simulink model "fil_videosharp_sim"  (R2018b)
settings: Solver=FixedStepDiscrete  StartTime=0.0  StopTime=inf  RelTol=1e-3
InitFcn:
  | filter = fi(fspecial('unsharp'),1,16,12);
  | 
  | % video size excluding the blanking periods
  | fileName = get_param('fil_videosharp_sim/From Multimedia File',  'inputFilename');
  | x=mmfileinfo(fileName);
  | v = x.Video ;
  | H = v.Height;
  | W = v.Width;
  | %H = 176;
  | %W = 240;
  | activeVideoSize = [H W];
  | 
  | % horizontal and vertical blanking
  | hBlanking = 0;
  | vBlanking = 0;
undefined symbols (not defined in the file): gcbh, gray, none, NumBits1, NumBits2, Rec, SDTV, Slope1, Slope2, videoinput
libraries: simulink x19, visionconversions x3, dspsigattribs x3, visiongeotforms x3, dspbuff3 x3, hdlsllib x3, visionsinks x1, dspvision x1, imaqlib x1, simulink_need_slupdate x1, fillib x1
(part 3 of 3)

== system fil_videosharp_sim/Streaming 2-D FIR Filter/Line Memory/Line Memory Controller/Write Col Counter ==
  enable : Inport
  reload : Inport  Port=2
  DataTypeConversion : DataTypeConversion  OutDataTypeStr=fixdt(SIGN==1,((WLTYPE==1) * ( ceil(log2(MAX_VAL-MIN_VAL+1)) + double(SIGN==1) ) ) + ((WLTYPE~=1)* WL ),0)
  Unit Delay : UnitDelay  InitialCondition=INIT_VAL  SampleTime=-1
  eML Counter : MATLAB Function  TreatAsAtomicUnit=on
  count : Outport
  wires:
  DataTypeConversion/1 -> Unit Delay/1
  eML Counter/1(nextCount) -> DataTypeConversion/1
  Unit Delay/1 -> eML Counter/1(currentCount), count/1
  reload/1 -> eML Counter/3(reload)
  enable/1 -> eML Counter/2(enb)

== system fil_videosharp_sim/Streaming 2-D FIR Filter/Line Memory/Line Memory Controller/Write Line Counter ==
  enable : Inport
  reload : Inport  Port=2
  DataTypeConversion : DataTypeConversion  OutDataTypeStr=fixdt(SIGN==1,((WLTYPE==1) * ( ceil(log2(MAX_VAL-MIN_VAL+1)) + double(SIGN==1) ) ) + ((WLTYPE~=1)* WL ),0)
  Unit Delay : UnitDelay  InitialCondition=INIT_VAL  SampleTime=-1
  eML Counter : MATLAB Function  TreatAsAtomicUnit=on
  count : Outport
  wires:
  enable/1 -> eML Counter/2(enb)
  reload/1 -> eML Counter/3(reload)
  Unit Delay/1 -> eML Counter/1(currentCount), count/1
  eML Counter/1(nextCount) -> DataTypeConversion/1
  DataTypeConversion/1 -> Unit Delay/1

== system fil_videosharp_sim/Streaming 2-D FIR Filter/Line Memory/Line Memory Controller/zzzz1 ==

== system fil_videosharp_sim/Streaming 2-D FIR Filter/Line Memory/Line Memory Controller/zzzz3 ==

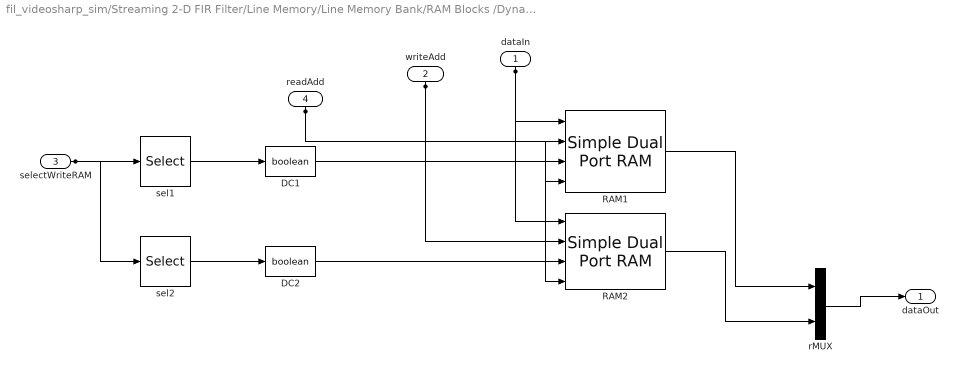
== system fil_videosharp_sim/Streaming 2-D FIR Filter/Line Memory/Line Memory Bank/RAM Blocks /Dynamic RAM Blocks ==
  dataIn : Inport
  writeAdd : Inport  Port=2
  selectWriteRAM : Inport  Port=3
  readAdd : Inport  Port=4
  DC1 : DataTypeConversion  OutDataTypeStr=boolean
  DC2 : DataTypeConversion  OutDataTypeStr=boolean
  RAM1 : hdlsllib/HDL RAMs/Simple Dual Port RAM  ram_size=WL
      settings: SourceProductName=HDL Coder  SourceProductBaseCode=HD
  RAM2 : hdlsllib/HDL RAMs/Simple Dual Port RAM  ram_size=WL
      settings: SourceProductName=HDL Coder  SourceProductBaseCode=HD
  rMUX : Mux  Inputs=2
  sel1 : Selector  InputPortWidth=2  IndexOptions=Index vector (dialog)  Indices=[1]  OutputSizes=1
  sel2 : Selector  InputPortWidth=2  IndexOptions=Index vector (dialog)  Indices=[2]  OutputSizes=1
  dataOut : Outport
  wires:
  selectWriteRAM/1 -> sel1/1, sel2/1
  sel1/1 -> DC1/1
  DC1/1 -> RAM1/3
  dataIn/1 -> RAM1/1, RAM2/1
  writeAdd/1 -> RAM1/2, RAM2/2
  readAdd/1 -> RAM1/4, RAM2/4
  RAM1/1 -> rMUX/1
  sel2/1 -> DC2/1
  DC2/1 -> RAM2/3
  RAM2/1 -> rMUX/2
  rMUX/1 -> dataOut/1

== system fil_videosharp_sim/Streaming 2-D FIR Filter/Line Memory/Line Memory Controller/Adjust Sync Signals/Detect Frame End ==
  lineEnd : Inport
  frameHeight : Inport  Port=2
  rowIndex : Inport  Port=3
  AND1 : Logic  IconShape=distinctive  AllPortsSameDT=off  OutDataTypeStr=boolean
  Add : Sum
  Constant2 : Constant  OutDataTypeStr=Inherit: Inherit via back propagation
  Relational Operator : RelationalOperator  Operator===  OutDataTypeStr=boolean  RndMeth=Nearest
  valid : Outport
  wires:
  Constant2/1 -> Add/1
  Add/1 -> Relational Operator/2
  Relational Operator/1 -> AND1/2
  lineEnd/1 -> AND1/1
  rowIndex/1 -> Add/2
  frameHeight/1 -> Relational Operator/1
  AND1/1 -> valid/1

== system fil_videosharp_sim/Streaming 2-D FIR Filter/Line Memory/Line Memory Controller/Adjust Sync Signals/Detect Frame Start ==
  lineStart : Inport
  rowIndex : Inport  Port=2
  AND1 : Logic  IconShape=distinctive  AllPortsSameDT=off  OutDataTypeStr=boolean
  Compare To Constant1 : simulink/Logic and Bit Operations/Compare To Constant  relop===  const=0  OutDataTypeStr=boolean  ZeroCross=off
  alignedFrameStart : Outport
  wires:
  AND1/1 -> alignedFrameStart/1
  rowIndex/1 -> Compare To Constant1/1
  lineStart/1 -> AND1/1
  Compare To Constant1/1 -> AND1/2

== system fil_videosharp_sim/Streaming 2-D FIR Filter/Line Memory/Line Memory Controller/Adjust Sync Signals/Detect Line End ==
  dataValidOut : Inport
  frameWidth : Inport  Port=2
  colIndex : Inport  Port=3
  AND1 : Logic  IconShape=distinctive  AllPortsSameDT=off  OutDataTypeStr=boolean
  Add : Sum
  Constant2 : Constant  OutDataTypeStr=Inherit: Inherit via back propagation
  Relational Operator : RelationalOperator  Operator===  OutDataTypeStr=boolean  RndMeth=Nearest
  lineEnd : Outport
  wires:
  AND1/1 -> lineEnd/1
  frameWidth/1 -> Relational Operator/1
  colIndex/1 -> Add/2
  dataValidOut/1 -> AND1/1
  Relational Operator/1 -> AND1/2
  Add/1 -> Relational Operator/2
  Constant2/1 -> Add/1

== system fil_videosharp_sim/Streaming 2-D FIR Filter/Line Memory/Line Memory Controller/Adjust Sync Signals/Detect Line Start ==
  dataValidOut : Inport
  colIndex : Inport  Port=2
  AND1 : Logic  AllPortsSameDT=off  OutDataTypeStr=boolean
  Compare To Constant1 : simulink/Logic and Bit Operations/Compare To Constant  relop===  const=0  OutDataTypeStr=boolean  ZeroCross=off
  alignedLineStart : Outport
  wires:
  Compare To Constant1/1 -> AND1/2
  dataValidOut/1 -> AND1/1
  colIndex/1 -> Compare To Constant1/1
  AND1/1 -> alignedLineStart/1

== system fil_videosharp_sim/Streaming 2-D FIR Filter/Line Memory/Line Memory Controller/Adjust Sync Signals/SyncMux ==
  activePixel : Inport
  lineStart : Inport  Port=2
  lineEnd : Inport  Port=3
  FrameStart : Inport  Port=4
  FrameEnd : Inport  Port=5
  Mux : Mux  Inputs=5
  syncOut : Outport
  wires:
  Mux/1 -> syncOut/1
  FrameEnd/1 -> Mux/5
  FrameStart/1 -> Mux/4
  lineEnd/1 -> Mux/3
  lineStart/1 -> Mux/2
  activePixel/1 -> Mux/1

== system fil_videosharp_sim/Streaming 2-D FIR Filter/Line Memory/Line Memory Controller/Read Control/Hold Valid Counter ==
  enable : Inport
  reload : Inport  Port=2
  DataTypeConversion : DataTypeConversion  OutDataTypeStr=fixdt(SIGN==1,((WLTYPE==1) * ( ceil(log2(MAX_VAL-MIN_VAL+1)) + double(SIGN==1) ) ) + ((WLTYPE~=1)* WL ),0)
  Unit Delay : UnitDelay  InitialCondition=INIT_VAL  SampleTime=-1
  eML Counter : MATLAB Function  TreatAsAtomicUnit=on
  count : Outport
  wires:
  enable/1 -> eML Counter/2(enb)
  reload/1 -> eML Counter/3(reload)
  Unit Delay/1 -> eML Counter/1(currentCount), count/1
  eML Counter/1(nextCount) -> DataTypeConversion/1
  DataTypeConversion/1 -> Unit Delay/1

== system fil_videosharp_sim/Streaming 2-D FIR Filter/Line Memory/Line Memory Controller/Read Control/Pos Edge Detect ==
  x : Inport
  Logical Operator1 : Logic  AllPortsSameDT=off  OutDataTypeStr=boolean
  Logical Operator2 : Logic  Operator=NOT  AllPortsSameDT=off  OutDataTypeStr=boolean
  Unit Delay1 : UnitDelay  SampleTime=-1
  y : Outport
  wires:
  x/1 -> Logical Operator1/1, Unit Delay1/1
  Logical Operator1/1 -> y/1
  Logical Operator2/1 -> Logical Operator1/2
  Unit Delay1/1 -> Logical Operator2/1

== system fil_videosharp_sim/Streaming 2-D FIR Filter/Line Memory/Line Memory Controller/Read Control/Pos Edge Detect1 ==
  x : Inport
  Logical Operator1 : Logic  AllPortsSameDT=off  OutDataTypeStr=boolean
  Logical Operator2 : Logic  Operator=NOT  AllPortsSameDT=off  OutDataTypeStr=boolean
  Unit Delay1 : UnitDelay  SampleTime=-1
  y : Outport
  wires:
  x/1 -> Logical Operator1/1, Unit Delay1/1
  Logical Operator1/1 -> y/1
  Logical Operator2/1 -> Logical Operator1/2
  Unit Delay1/1 -> Logical Operator2/1

== system fil_videosharp_sim/Streaming 2-D FIR Filter/Line Memory/Line Memory Controller/Read Control/Repeat Counter ==
  enable : Inport
  reload : Inport  Port=2
  DataTypeConversion : DataTypeConversion  OutDataTypeStr=fixdt(SIGN==1,((WLTYPE==1) * ( ceil(log2(MAX_VAL-MIN_VAL+1)) + double(SIGN==1) ) ) + ((WLTYPE~=1)* WL ),0)
  Unit Delay : UnitDelay  InitialCondition=INIT_VAL  SampleTime=-1
  eML Counter : MATLAB Function  TreatAsAtomicUnit=on
  count : Outport
  wires:
  DataTypeConversion/1 -> Unit Delay/1
  eML Counter/1(nextCount) -> DataTypeConversion/1
  Unit Delay/1 -> eML Counter/1(currentCount), count/1
  reload/1 -> eML Counter/3(reload)
  enable/1 -> eML Counter/2(enb)

== system fil_videosharp_sim/Streaming 2-D FIR Filter/Line Memory/Line Memory Controller/Read Control/Time Distance ==
  repeat : Inport
  newLine : Inport  Port=2
  Time Distance : MATLAB Function  TreatAsAtomicUnit=on
  Unit Delay1 : UnitDelay  SampleTime=-1
  Unit Delay7 : UnitDelay  SampleTime=-1
  currentDistance : Outport
  lastDistance : Outport  Port=2
  wires:
  repeat/1 -> Time Distance/2(repeatPulse)
  Unit Delay1/1 -> Time Distance/4(fromLastDist), lastDistance/1
  Unit Delay7/1 -> Time Distance/3(fromDistCounter), currentDistance/1
  newLine/1 -> Time Distance/1(inputPulse)
  Time Distance/2(toLastDist) -> Unit Delay1/1  "current_dist"
  Time Distance/1(toDistCounter) -> Unit Delay7/1  "Last_dist"

== system fil_videosharp_sim/Streaming 2-D FIR Filter/Line Memory/Line Memory Controller/Read Control/zzzz1 ==

== system fil_videosharp_sim/Streaming 2-D FIR Filter/Line Memory/Line Memory Controller/Read Control/zzzz2 ==

== system fil_videosharp_sim/Streaming 2-D FIR Filter/Line Memory/Line Memory Controller/Read Control/zzzz3 ==

== system fil_videosharp_sim/Streaming 2-D FIR Filter/Line Memory/Line Memory Controller/Read Control/zzzz5 ==

== system fil_videosharp_sim/Streaming 2-D FIR Filter/Line Memory/Line Memory Controller/Read Line Count/Read Line Counter1 ==
  enable : Inport
  reload : Inport  Port=2
  loadVal : Inport  Port=3
  DataTypeConversion : DataTypeConversion  OutDataTypeStr=fixdt(SIGN==1,((WLTYPE==1) * ( ceil(log2(MAX_VAL-MIN_VAL+1)) + double(SIGN==1) ) ) + ((WLTYPE~=1)* WL ),0)
  Unit Delay : UnitDelay  InitialCondition=INIT_VAL  SampleTime=-1
  eML Counter : MATLAB Function  TreatAsAtomicUnit=on
  count : Outport
  wires:
  enable/1 -> eML Counter/2(enb)
  reload/1 -> eML Counter/3(reload)
  Unit Delay/1 -> eML Counter/1(currentCount), count/1
  eML Counter/1(nextCount) -> DataTypeConversion/1
  DataTypeConversion/1 -> Unit Delay/1
  loadVal/1 -> eML Counter/4(loadVal)

== matlab function fil_videosharp_sim/Frame to Stream/Produce Row-Major Organized Output (Dimensions will be flipped) ==
  data: u input; y output; isInputRowMajor parameter
function y = condTranspose(u, isInputRowMajor)
%#eml

if (isInputRowMajor)
    y = u;
else
    y = permute(u,[2,1]);
end

== matlab function fil_videosharp_sim/Streaming 2-D FIR Filter/Line Memory/Aligned Demux/Aligned Pulse ==
  settings: fimath=hdlfimath
  data: valid input; earlyPulse input; alignedPulse output
function alignedPulse = align(valid,earlyPulse)

persistent earlyPulse_reg;
if isempty(earlyPulse_reg)
    earlyPulse_reg = false;
end

alignedPulse= (earlyPulse_reg || earlyPulse) && valid;

if (earlyPulse && ~valid)
    earlyPulse_reg=true;
elseif (earlyPulse_reg || earlyPulse) && valid;
    earlyPulse_reg=false;
end

== matlab function fil_videosharp_sim/Stream to Frame/Generate Control Signals ==
  data: activePixel input; frameValid output; frameStart input; frameEnd input; enable output
function [frameValid, enable] = ctrlSigGen(activePixel, frameStart, ...
    frameEnd)
%#eml

persistent enableFlag; % turns on after vsync pulse was received

persistent frameEndWithDelay;

% initialize persistent vars
if isempty(enableFlag)
   enableFlag = false; 
end

if isempty(frameEndWithDelay)
   frameEndWithDelay = false; 
end

if frameStart ~= 0
    enableFlag = true;
end

enable = frameEndWithDelay || activePixel;

frameValid =  frameEndWithDelay;


% Delay line block used to accumulate full frame has an inherent
% latency of 1.  We accommodate it by using a delayed version of 
% frameEnd signal in computing the enableFlag
frameEndWithDelay = frameEnd;

== matlab function fil_videosharp_sim/Frame to Stream/Generate Control Signals ==
  data: unused input; sync output; activeVideo input; hBlanking parameter; vBlanking parameter
% This function generates synchronization signals:
% [activePixels, lineStart, lineEnd, frameStart, frameEnd]

function sync  = ctrlSigGen(~, activeVideo, hBlanking, vBlanking)
% Note: the first unsed variable is fed into this function purely for
%       the purpose of establishing a rate that will be used by this
%       EML block; we don't want to rely on the back-propagated rate since
%       this approach is more robust

%#eml

persistent numActivePixels;
persistent videoIdx;
persistent countForFrameSkip;

if isempty(numActivePixels) % initialize only once
    numActivePixels   = 0;
    videoIdx          = 1;
    countForFrameSkip = 0;
end

% extract various information about the input video stream
activeVideoSize  = size(activeVideo);
activeVideoNumel = prod(activeVideoSize);
activeVideoWidth = activeVideoSize(2);

videoSize  = activeVideoSize + [vBlanking hBlanking];
videoNumel = prod(videoSize);

% Unbuffer block has a latency of one frame; start sending sync 
% signals after one frame is accumulated in the delay line
if countForFrameSkip <  videoNumel
    countForFrameSkip = countForFrameSkip + 1;
    sync = false(5,1); % sync signals are disabled
    return;
end

% Upper left corner of active video is situated at [0 hBlanking] location,
% while lower right corner of active video is at [activeVideoSize(1) 
% videoSize(2)]
modOfWidth = mod(videoIdx, videoSize(2));
isActivePixel = ((modOfWidth > hBlanking) || ~modOfWidth ) && ...
    (videoIdx <= videoSize(2)*activeVideoSize(1));

% generate the remainder of sync signals
if isActivePixel % only check upon arrival of new active pixel
    numActivePixels = numActivePixels + 1;
    
    lineStart  = (mod(numActivePixels, activeVideoWidth) == 1);
    lineEnd    = ~mod(numActivePixels, activeVideoWidth);    
    frameStart = (numActivePixels == 1);
    frameEnd   = (numActivePixels == activeVideoNumel);
else
    lineStart  = false; lineEnd  = false; 
    frameStart = false; frameEnd = false;
end

% move to the next location in the mask
videoIdx = videoIdx+1;
% reset videoIdx counter
if videoIdx == videoNumel+1
    videoIdx = 1;
end

% reset the numActivePixels count
if frameEnd
    numActivePixels = 0;
end

sync = [isActivePixel,lineStart,lineEnd,frameStart,frameEnd]';

== matlab function fil_videosharp_sim/Streaming 2-D FIR Filter/Line Memory/Aligned Demux/Aligned Pulse1 ==
  settings: fimath=hdlfimath
  data: valid input; earlyPulse input; alignedPulse output
function alignedPulse = align(valid,earlyPulse)

persistent earlyPulse_reg;
if isempty(earlyPulse_reg)
    earlyPulse_reg = false;
end

alignedPulse= (earlyPulse_reg || earlyPulse) && valid;

if (earlyPulse && ~valid)
    earlyPulse_reg=true;
elseif (earlyPulse_reg || earlyPulse) && valid;
    earlyPulse_reg=false;
end

== matlab function fil_videosharp_sim/Streaming 2-D FIR Filter/Line Memory/Line Memory Bank/Line Selector ==
  data: selectReadLine input; inputLines input; latestPixel input; y output
function y = line_selector(selectReadLine,inputLines,latestPixel)

if isfi(inputLines)
    nt = numerictype(inputLines(1));
else
    nt = numerictype(class(inputLines));
end

selected_lines = fi(zeros(length(inputLines)+1,1),nt);
 
for i= 1:length(inputLines)
    selected_lines(i) = inputLines(int(selectReadLine(i))+1); 
end

selected_lines(length(inputLines)+1) = latestPixel;
y = selected_lines;

== matlab function fil_videosharp_sim/Streaming 2-D FIR Filter/Line Memory/Line Memory Bank/decoder ==
  data: selectWriteLine input; writeValid input; y output; nL parameter
function y = decoder(selectWriteLine,writeValid,nL)

decoded = fi(zeros(nL-1,1),0,1,0);

for i= 1:nL-1
    swl = int(selectWriteLine); 
    if swl==(i-1) && writeValid
        decoded(i)= fi(1,0,1,0);
    else 
        decoded(i)= fi(0,0,1,0);
    end        
end

y = decoded;

== matlab function fil_videosharp_sim/Streaming 2-D FIR Filter/Line Memory/Line Memory Controller/Initial Line Skip/eML Counter ==
  data: currentCount input; enb input; nextCount output; reload input; INIT_VAL parameter; STEP_VAL parameter; MIN_VAL parameter; MAX_VAL parameter; RELOADTYPE parameter; RELOAD_VAL parameter; STOPTYPE parameter; STOP_VAL parameter; ROLLTYPE parameter; ROLL_VAL parameter; SIGN parameter; WLTYPE parameter; WL parameter
function nextCount = couner(currentCount,enb,reload,INIT_VAL,STEP_VAL,MIN_VAL,MAX_VAL,...
    RELOADTYPE,RELOAD_VAL,STOPTYPE,STOP_VAL,ROLLTYPE,ROLL_VAL,...
    SIGN,WLTYPE,WL)
%#eml

if (SIGN==1) 
    sign=1;
else
    sign =0;
end
if (WLTYPE==1)
    wl = ceil(log2(MAX_VAL-MIN_VAL+1)) + sign ;
else 
    wl= WL;
end


if STOPTYPE==1
    stop=false;
else
    stop=true; 
end
stop_val= STOP_VAL;

if RELOADTYPE==1
    reload_val = INIT_VAL;
else 
    reload_val = RELOAD_VAL;
end
if ROLLTYPE==1
    roll_val=INIT_VAL;
else 
    roll_val=ROLL_VAL;
end


if reload 
    nextCount = fi(reload_val,sign,wl,0);
else 
    if enb
        if (STEP_VAL>0  && (int(currentCount)+STEP_VAL)<= stop_val) || (STEP_VAL<=0 && (int(currentCount)+STEP_VAL)>= stop_val)
            nextCount=fi(int(currentCount)+STEP_VAL,sign,wl,0);
        else
            if stop
                nextCount=fi(int(currentCount),sign,wl,0);
            else 
                nextCount=fi(roll_val,sign,wl,0);
            end
        end            
    else
      nextCount=fi(int(currentCount),sign,wl,0); 
    end
end

== matlab function fil_videosharp_sim/Streaming 2-D FIR Filter/Line Memory/Line Memory Controller/Out Row Count/eML Counter ==
  data: currentCount input; enb input; nextCount output; reload input; INIT_VAL parameter; STEP_VAL parameter; MIN_VAL parameter; MAX_VAL parameter; RELOADTYPE parameter; RELOAD_VAL parameter; STOPTYPE parameter; STOP_VAL parameter; ROLLTYPE parameter; ROLL_VAL parameter; SIGN parameter; WLTYPE parameter; WL parameter
function nextCount = couner(currentCount,enb,reload,INIT_VAL,STEP_VAL,MIN_VAL,MAX_VAL,...
    RELOADTYPE,RELOAD_VAL,STOPTYPE,STOP_VAL,ROLLTYPE,ROLL_VAL,...
    SIGN,WLTYPE,WL)
%#eml

if (SIGN==1) 
    sign=1;
else
    sign =0;
end
if (WLTYPE==1)
    wl = ceil(log2(MAX_VAL-MIN_VAL+1)) + sign ;
else 
    wl= WL;
end


if STOPTYPE==1
    stop=false;
else
    stop=true; 
end
stop_val= STOP_VAL;

if RELOADTYPE==1
    reload_val = INIT_VAL;
else 
    reload_val = RELOAD_VAL;
end
if ROLLTYPE==1
    roll_val=INIT_VAL;
else 
    roll_val=ROLL_VAL;
end


if reload 
    nextCount = fi(reload_val,sign,wl,0);
else 
    if enb
        if (STEP_VAL>0  && (int(currentCount)+STEP_VAL)<= stop_val) || (STEP_VAL<=0 && (int(currentCount)+STEP_VAL)>= stop_val)
            nextCount=fi(int(currentCount)+STEP_VAL,sign,wl,0);
        else
            if stop
                nextCount=fi(int(currentCount),sign,wl,0);
            else 
                nextCount=fi(roll_val,sign,wl,0);
            end
        end            
    else
      nextCount=fi(int(currentCount),sign,wl,0); 
    end
end

== matlab function fil_videosharp_sim/Streaming 2-D FIR Filter/Line Memory/Line Memory Controller/Read Col Counter/eML Counter ==
  data: currentCount input; enb input; nextCount output; reload input; INIT_VAL parameter; STEP_VAL parameter; MIN_VAL parameter; MAX_VAL parameter; RELOADTYPE parameter; RELOAD_VAL parameter; STOPTYPE parameter; STOP_VAL parameter; ROLLTYPE parameter; ROLL_VAL parameter; SIGN parameter; WLTYPE parameter; WL parameter
function nextCount = counter(currentCount,enb,reload,INIT_VAL,STEP_VAL,MIN_VAL,MAX_VAL,...
    RELOADTYPE,RELOAD_VAL,STOPTYPE,STOP_VAL,ROLLTYPE,ROLL_VAL,...
    SIGN,WLTYPE,WL)
%#eml

if (SIGN==1) 
    sign=1;
else
    sign =0;
end
if (WLTYPE==1)
    wl = ceil(log2(MAX_VAL-MIN_VAL+1)) + sign ;
else 
    wl= WL;
end


if STOPTYPE==1
    stop=false;
else
    stop=true; 
end
stop_val= STOP_VAL;

if RELOADTYPE==1
    reload_val = INIT_VAL;
else 
    reload_val = RELOAD_VAL;
end
if ROLLTYPE==1
    roll_val=INIT_VAL;
else 
    roll_val=ROLL_VAL;
end


if reload 
    nextCount = fi(reload_val,sign,wl,0);
else 
    if enb
        if (STEP_VAL>0  && (int(currentCount)+STEP_VAL)<= stop_val) || (STEP_VAL<=0 && (int(currentCount)+STEP_VAL)>= stop_val)
            nextCount=fi(int(currentCount)+STEP_VAL,sign,wl,0);
        else
            if stop
                nextCount=fi(int(currentCount),sign,wl,0);
            else 
                nextCount=fi(roll_val,sign,wl,0);
            end
        end            
    else
      nextCount=fi(int(currentCount),sign,wl,0); 
    end
end

== matlab function fil_videosharp_sim/Streaming 2-D FIR Filter/Line Memory/Line Memory Controller/Read Control/Aligned to Second Pulse ==
  settings: fimath=hdlfimath
  data: earlyPulse input; latePulse input; out output
function out = wait_for_two_pulse(earlyPulse,latePulse)

persistent early_pulse_reg;
if isempty(early_pulse_reg)
    early_pulse_reg = false;
end

out= (early_pulse_reg || earlyPulse) && latePulse;

if (earlyPulse && ~latePulse)
    early_pulse_reg=true;
elseif (early_pulse_reg || earlyPulse) && latePulse;
    early_pulse_reg=false;

end

== matlab function fil_videosharp_sim/Streaming 2-D FIR Filter/Line Memory/Line Memory Controller/Read Control/Bit Set ==
  settings: fimath=hdlfimath
  data: set input; status output; reset input
function status = f(set,reset)

persistent status_reg;
if isempty(status_reg)
    status_reg =false;
end

status = status_reg ;

if set 
    status_reg = true;
elseif reset
    status_reg= false;
end

== matlab function fil_videosharp_sim/Streaming 2-D FIR Filter/Line Memory/Line Memory Controller/Read Control/Hold Valid Counter/eML Counter ==
  data: currentCount input; enb input; nextCount output; reload input; INIT_VAL parameter; STEP_VAL parameter; MIN_VAL parameter; MAX_VAL parameter; RELOADTYPE parameter; RELOAD_VAL parameter; STOPTYPE parameter; STOP_VAL parameter; ROLLTYPE parameter; ROLL_VAL parameter; SIGN parameter; WLTYPE parameter; WL parameter
function nextCount = couner(currentCount,enb,reload,INIT_VAL,STEP_VAL,MIN_VAL,MAX_VAL,...
    RELOADTYPE,RELOAD_VAL,STOPTYPE,STOP_VAL,ROLLTYPE,ROLL_VAL,...
    SIGN,WLTYPE,WL)
%#eml

if (SIGN==1) 
    sign=1;
else
    sign =0;
end
if (WLTYPE==1)
    wl = ceil(log2(MAX_VAL-MIN_VAL+1)) + sign ;
else 
    wl= WL;
end


if STOPTYPE==1
    stop=false;
else
    stop=true; 
end
stop_val= STOP_VAL;

if RELOADTYPE==1
    reload_val = INIT_VAL;
else 
    reload_val = RELOAD_VAL;
end
if ROLLTYPE==1
    roll_val=INIT_VAL;
else 
    roll_val=ROLL_VAL;
end


if reload 
    nextCount = fi(reload_val,sign,wl,0);
else 
    if enb
        if (STEP_VAL>0  && (int(currentCount)+STEP_VAL)<= stop_val) || (STEP_VAL<=0 && (int(currentCount)+STEP_VAL)>= stop_val)
            nextCount=fi(int(currentCount)+STEP_VAL,sign,wl,0);
        else
            if stop
                nextCount=fi(int(currentCount),sign,wl,0);
            else 
                nextCount=fi(roll_val,sign,wl,0);
            end
        end            
    else
      nextCount=fi(int(currentCount),sign,wl,0); 
    end
end

== matlab function fil_videosharp_sim/Streaming 2-D FIR Filter/Line Memory/Line Memory Controller/Read Control/Repeat Counter/eML Counter ==
  data: currentCount input; enb input; nextCount output; reload input; INIT_VAL parameter; STEP_VAL parameter; MIN_VAL parameter; MAX_VAL parameter; RELOADTYPE parameter; RELOAD_VAL parameter; STOPTYPE parameter; STOP_VAL parameter; ROLLTYPE parameter; ROLL_VAL parameter; SIGN parameter; WLTYPE parameter; WL parameter
function nextCount = couner(currentCount,enb,reload,INIT_VAL,STEP_VAL,MIN_VAL,MAX_VAL,...
    RELOADTYPE,RELOAD_VAL,STOPTYPE,STOP_VAL,ROLLTYPE,ROLL_VAL,...
    SIGN,WLTYPE,WL)
%#eml

if (SIGN==1) 
    sign=1;
else
    sign =0;
end
if (WLTYPE==1)
    wl = ceil(log2(MAX_VAL-MIN_VAL+1)) + sign ;
else 
    wl= WL;
end


if STOPTYPE==1
    stop=false;
else
    stop=true; 
end
stop_val= STOP_VAL;

if RELOADTYPE==1
    reload_val = INIT_VAL;
else 
    reload_val = RELOAD_VAL;
end
if ROLLTYPE==1
    roll_val=INIT_VAL;
else 
    roll_val=ROLL_VAL;
end


if reload 
    nextCount = fi(reload_val,sign,wl,0);
else 
    if enb
        if (STEP_VAL>0  && (int(currentCount)+STEP_VAL)<= stop_val) || (STEP_VAL<=0 && (int(currentCount)+STEP_VAL)>= stop_val)
            nextCount=fi(int(currentCount)+STEP_VAL,sign,wl,0);
        else
            if stop
                nextCount=fi(int(currentCount),sign,wl,0);
            else 
                nextCount=fi(roll_val,sign,wl,0);
            end
        end            
    else
      nextCount=fi(int(currentCount),sign,wl,0); 
    end
end

== matlab function fil_videosharp_sim/Streaming 2-D FIR Filter/Line Memory/Line Memory Controller/Read Control/Time Distance/Time Distance ==
  settings: fimath=hdlfimath
  data: inputPulse input; repeatPulse input; fromDistCounter input fixdt(0,ceil(log2(2*maxnc +1)),0); fromLastDist input fixdt(0,ceil(log2(2*maxnc +1)),0); toDistCounter output; maxnc parameter; toLastDist output
function [toDistCounter,toLastDist] = ...
    time_distance(inputPulse,repeatPulse,...
    fromDistCounter,fromLastDist,maxnc)

WL = ceil(log2(2*maxnc +1));
%WL = 8;

if inputPulse || repeatPulse
    if inputPulse
        toLastDist = fromDistCounter;
    else
         toLastDist = fromLastDist;
    end
    toDistCounter = fi(1,0,WL,0);
else 
      if int(fromDistCounter) < 2*maxnc 
          toDistCounter =  fi( int(fromDistCounter)+1,0,WL,0);
      else
          toDistCounter = fromDistCounter;
      end
      toLastDist = fromLastDist;
end

== matlab function fil_videosharp_sim/Streaming 2-D FIR Filter/Line Memory/Line Memory Controller/Read Line Count/Read Line Counter1/eML Counter ==
  data: currentCount input; enb input; nextCount output; reload input; loadVal input; INIT_VAL parameter; STEP_VAL parameter; MIN_VAL parameter; MAX_VAL parameter; RELOADTYPE parameter; RELOAD_VAL parameter; STOPTYPE parameter; STOP_VAL parameter; ROLLTYPE parameter; ROLL_VAL parameter; SIGN parameter; WLTYPE parameter; WL parameter
function nextCount = couner(currentCount,enb,reload,loadVal,INIT_VAL,STEP_VAL,MIN_VAL,MAX_VAL,...
    RELOADTYPE,RELOAD_VAL,STOPTYPE,STOP_VAL,ROLLTYPE,ROLL_VAL,...
    SIGN,WLTYPE,WL)
%#eml

if (SIGN==1) 
    sign=1;
else
    sign =0;
end
if (WLTYPE==1)
    wl = ceil(log2(MAX_VAL-MIN_VAL+1)) + sign ;
else 
    wl= WL;
end


if STOPTYPE==1
    stop=false;
else
    stop=true; 
end
stop_val= STOP_VAL;

% if RELOADTYPE==1
%     reload_val = INIT_VAL;
% else 
%     reload_val = RELOAD_VAL;
% end

reload_val = loadVal;
if ROLLTYPE==1
    roll_val=INIT_VAL;
else 
    roll_val=ROLL_VAL;
end


if reload 
    nextCount = fi(reload_val,sign,wl,0);
else 
    if enb
        if (STEP_VAL>0  && (int(currentCount)+STEP_VAL)<= stop_val) || (STEP_VAL<=0 && (int(currentCount)+STEP_VAL)>= stop_val)
            nextCount=fi(int(currentCount)+STEP_VAL,sign,wl,0);
        else
            if stop
                nextCount=fi(int(currentCount),sign,wl,0);
            else 
                nextCount=fi(roll_val,sign,wl,0);
            end
        end            
    else
      nextCount=fi(int(currentCount),sign,wl,0); 
    end
end

== matlab function fil_videosharp_sim/Streaming 2-D FIR Filter/Line Memory/Line Memory Controller/Select All Output Rows ==
  data: readLineCount input; y output; nL parameter
function y = fcn(readLineCount,nL)

reverse_index=nL-2:-1:0;

% output word-length
owl = ceil(log2(nL-1)); 
if (owl <= 0 ) 
    OWL =1;
else
    OWL =owl;
end

lut_vec=fi(zeros(nL-1,nL-1),0,OWL,0);
for k = 1:nL-1 
    out= fi(0:nL-2,0,OWL,0);
    for i=0:nL-2   
        j= i-(nL-k);
        if (j) <0 
            out(i+1)= fi(reverse_index(-j),0,OWL,0);
        else
            out(i+1)=fi(j,0,OWL,0);
        end        
    end
    lut_vec(:,k)= out;
end

out_vec = fi(zeros(nL-1,1),0,OWL,0);

lut_r=int(readLineCount)+1;  

for i=1:nL-1
    fx_lut_ele = fi(lut_vec(lut_r,i),0,OWL,0);
    out_vec(i) = fx_lut_ele; 
end
y = out_vec;

== matlab function fil_videosharp_sim/Streaming 2-D FIR Filter/Line Memory/Line Memory Controller/Write Col Counter/eML Counter ==
  data: currentCount input; enb input; nextCount output; reload input; INIT_VAL parameter; STEP_VAL parameter; MIN_VAL parameter; MAX_VAL parameter; RELOADTYPE parameter; RELOAD_VAL parameter; STOPTYPE parameter; STOP_VAL parameter; ROLLTYPE parameter; ROLL_VAL parameter; SIGN parameter; WLTYPE parameter; WL parameter
function nextCount = couner(currentCount,enb,reload,INIT_VAL,STEP_VAL,MIN_VAL,MAX_VAL,...
    RELOADTYPE,RELOAD_VAL,STOPTYPE,STOP_VAL,ROLLTYPE,ROLL_VAL,...
    SIGN,WLTYPE,WL)
%#eml

if (SIGN==1) 
    sign=1;
else
    sign =0;
end
if (WLTYPE==1)
    wl = ceil(log2(MAX_VAL-MIN_VAL+1)) + sign ;
else 
    wl= WL;
end


if STOPTYPE==1
    stop=false;
else
    stop=true; 
end
stop_val= STOP_VAL;

if RELOADTYPE==1
    reload_val = INIT_VAL;
else 
    reload_val = RELOAD_VAL;
end
if ROLLTYPE==1
    roll_val=INIT_VAL;
else 
    roll_val=ROLL_VAL;
end


if reload 
    nextCount = fi(reload_val,sign,wl,0);
else 
    if enb
        if (STEP_VAL>0  && (int(currentCount)+STEP_VAL)<= stop_val) || (STEP_VAL<=0 && (int(currentCount)+STEP_VAL)>= stop_val)
            nextCount=fi(int(currentCount)+STEP_VAL,sign,wl,0);
        else
            if stop
                nextCount=fi(int(currentCount),sign,wl,0);
            else 
                nextCount=fi(roll_val,sign,wl,0);
            end
        end            
    else
      nextCount=fi(int(currentCount),sign,wl,0); 
    end
end

== matlab function fil_videosharp_sim/Streaming 2-D FIR Filter/Line Memory/Line Memory Controller/Write Line Counter/eML Counter ==
  data: currentCount input; enb input; nextCount output; reload input; INIT_VAL parameter; STEP_VAL parameter; MIN_VAL parameter; MAX_VAL parameter; RELOADTYPE parameter; RELOAD_VAL parameter; STOPTYPE parameter; STOP_VAL parameter; ROLLTYPE parameter; ROLL_VAL parameter; SIGN parameter; WLTYPE parameter; WL parameter
function nextCount = counter(currentCount,enb,reload,INIT_VAL,STEP_VAL,MIN_VAL,MAX_VAL,...
    RELOADTYPE,RELOAD_VAL,STOPTYPE,STOP_VAL,ROLLTYPE,ROLL_VAL,...
    SIGN,WLTYPE,WL)
%#eml

if (SIGN==1) 
    sign=1;
else
    sign =0;
end
if (WLTYPE==1)
    wl = ceil(log2(MAX_VAL-MIN_VAL+1)) + sign ;
else 
    wl= WL;
end


if STOPTYPE==1
    stop=false;
else
    stop=true; 
end
stop_val= STOP_VAL;

if RELOADTYPE==1
    reload_val = INIT_VAL;
else 
    reload_val = RELOAD_VAL;
end
if ROLLTYPE==1
    roll_val=INIT_VAL;
else 
    roll_val=ROLL_VAL;
end


if reload 
    nextCount = fi(reload_val,sign,wl,0);
else 
    if enb
        if (STEP_VAL>0  && (int(currentCount)+STEP_VAL)<= stop_val) || (STEP_VAL<=0 && (int(currentCount)+STEP_VAL)>= stop_val)
            nextCount=fi(int(currentCount)+STEP_VAL,sign,wl,0);
        else
            if stop
                nextCount=fi(int(currentCount),sign,wl,0);
            else 
                nextCount=fi(roll_val,sign,wl,0);
            end
        end            
    else
      nextCount=fi(int(currentCount),sign,wl,0); 
    end
end

== matlab function fil_videosharp_sim/Streaming 2-D FIR Filter/Make Neighborhood/Make Neighborhood ==
  data: columnIn input; colIndex input; rowIndex input; NH_ROWS parameter; NH_COLS parameter; frameSize input; OUTFORMAT parameter; PADDING parameter; PADVAL parameter; RIDXWL parameter; activePixel input; y output
function y = MakeNhood(columnIn,colIndex,rowIndex,NH_ROWS,NH_COLS,...
    frameSize,OUTFORMAT,PADDING,PADVAL,RIDXWL,activePixel)

%------------------- Algorithm description ---------------------
% 1. initialization 
%   1.1 shift registers  (for storing old data samples)
%   1.2 initial assignment for proper eML datatype  
%
% 2. column padding
%   2.1 counter declaration (count after last column)
%   2.2 boundary variables for column padding
%       2.2.1 head padding variables 
%       2.2.2 tail padding variables
%   2.3 padding action 
%
% 3. row padding 
%   3.1 declaration - row index register 
%   3.2 boundary variables for row padding
%       3.2.1 head padding variables 
%       3.2.2 tail padding variables
%   3.3 padding action
%
% 4. assign output 
%
% 5. updating persistent variables
%   5.1 shift registers (for storing old data_in)
%   5.2 row index register 
%   5.3 count after last column 
%-----------------------------------------------------------------
 
% ----------------------------------------------------------------
%                    1. initialization 
% ----------------------------------------------------------------
 
if isfi(columnIn)
    nt= numerictype(columnIn(1));
    ft = fimath(columnIn(1));
else
    nt = numerictype(class(columnIn));
    ft = fimath;
end
 
% ###  1.1 Shift registers  (for storing old data samples) ###
persistent old_cols;
if isempty(old_cols)
    old_cols = fi(zeros(NH_ROWS,NH_COLS-1), nt, ft);  
end

% ###  1.2 initial assignment for proper eML datatype ###
nhood = [old_cols columnIn ];
col_padded_nhood =  nhood;
row_padded_nhood =  col_padded_nhood;
 
% -----------------end  initialization ---------------------------
% ----------------------------------------------------------------
 
 
 
% ----------------------------------------------------------------
%                    2. column padding 
% ----------------------------------------------------------------
 
% ###  2.1 counter declaration ( count after last column)  ###
% We need a counter to  tell us how many clock cycles 
% has passed after we received a last column i.e. How deep 
% is the last column in the pipeline
persistent count_after_last_col;
max_calc_count = floor(NH_COLS/2);
if isempty(count_after_last_col)    
    count_WL= ceil(log2 (max_calc_count))+1;
    count_after_last_col =  fi(0,0,count_WL,0);
end

% ###   2.2 boundry variables for column Padding ###
 
% ###   2.2.1 head padding variables ###
start_col_head_pad = floor(NH_COLS/2); %start columns head padding 
                                       %when last column count is >= this 
stop_col_head_pad = NH_COLS-1; % stop columns head padding 
                                % when last column count > this
 
    % matrix indexes that needs to be padded
front_col_index = NH_COLS-int(colIndex);
%col_head_pad_from = 1; 
col_head_pad_until = front_col_index;
 
 
% ###  2.2.2 tail padding variables ### 
start_col_tail_pad = 1; % start columns tail padding 
                        % when count_after_last_col is >=this 
stop_col_tail_pad = max_calc_count; % stop columns tail padding 
                                    % when count_after_last_col is > this 
 
 
    % matrix indexes that needs to be padded
tail_col_index = NH_COLS-int(count_after_last_col);
col_tail_pad_from = tail_col_index;
%col_tail_pad_until = NH_COLS;
 
 
% ###   2.3 padding action ###
for i= 1:NH_COLS
    if i<col_head_pad_until && int(colIndex)>= start_col_head_pad ...
            && int(colIndex)<=stop_col_head_pad
        if PADDING==1 % zero padding
            col_padded_nhood(:,i)= fi(PADVAL*ones(NH_ROWS,1),nt,ft);
        elseif PADDING==2 % replicate padding
            col_padded_nhood(:,i)= nhood(:,front_col_index);
        else % mirror padding
            dist1 = front_col_index-i;
            col_padded_nhood(:,i)= nhood(:,front_col_index+dist1-1);
        end
    elseif i>col_tail_pad_from && ...
            int(count_after_last_col)>=start_col_tail_pad ...
            && int(count_after_last_col)<=stop_col_tail_pad
        if PADDING==1 % zero padding
            col_padded_nhood(:,i)= fi(PADVAL*ones(NH_ROWS,1),nt,ft);
        elseif PADDING==2 % replicate padding
            col_padded_nhood(:,i)= nhood(:,tail_col_index);
        else % mirror padding
            dist2 = (i-tail_col_index);
            col_padded_nhood(:,i)= nhood(:,tail_col_index-(dist2-1));
        end
    else
        col_padded_nhood(:,i)= nhood(:,i);
    end
end
% ----------------- end  column padding  -----------------------
% --------------------------------------------------------------
 
% ----------------------------------------------------------------
%                    3. Row padding 
% ----------------------------------------------------------------
 
% ###   3.1 declaration - row index register  ###
% the row index register will hold the value of the row index
% when the count after last column was zero
persistent row_index_reg;
%max_ridx_count = int(frameSize(1))+1;
if isempty(row_index_reg)
    count_WL = RIDXWL;
    %count_WL= ceil(log2 (max_ridx_count))+1;
    row_index_reg =  fi(0,0,count_WL,0);
end
% ###  3.2 boundary variables for row Padding  ###
 
% ###      3.2.1 head padding variables  ###
start_row_head_pad = 0; % start row head padding 
                        % when row index is >= this 
stop_row_head_pad = floor(NH_ROWS/2); % stop row head padding 
                                      % when row index > this
 
% matrix indexes that needs to be padded
front_row_index = ceil(NH_ROWS/2)-int(row_index_reg);
%row_head_pad_from = 1; 
row_head_pad_until = front_row_index;
 
% ###      3.2.2 tail padding variables  ###
start_row_tail_pad = int(frameSize(1))-floor(NH_ROWS/2); % start row tail padding
                                               % when row index is >= this 
stop_row_tail_pad = int(frameSize(1))-1; % stop row tail padding 
                               % when row index > this
 
 
 
% matrix indexes that needs to be padded
tail_row_index = int16(frameSize(1)) - int16(row_index_reg) +(ceil(NH_ROWS/2)-1); 
row_tail_pad_from = tail_row_index;
%row_tail_pad_until = NH_COLS;
 
% ###  3.3 padding action ###
for i= 1:NH_ROWS
       if i<row_head_pad_until && int(rowIndex)>= start_row_head_pad && ...
               int(rowIndex)<=stop_row_head_pad
           if PADDING==1 % zero padding 
               row_padded_nhood(i,:)= fi(PADVAL*ones(1,NH_COLS),nt,ft);
           elseif PADDING==2 % replicate padding
                row_padded_nhood(i,:)= col_padded_nhood(front_row_index,:); 
           else % mirror padding
               dist3 = (front_row_index-i);
               row_padded_nhood(i,:)= ...
                   col_padded_nhood(front_row_index+(dist3-1),:); 
           end
       elseif i>row_tail_pad_from && int(row_index_reg)>=start_row_tail_pad...
               && int(row_index_reg)<=stop_row_tail_pad
           if PADDING==1 % zero padding 
               row_padded_nhood(i,:)= fi(PADVAL*ones(1,NH_COLS),nt,ft);
           elseif PADDING==2 % replicate padding
               row_padded_nhood(i,:)= col_padded_nhood(tail_row_index,:);
           else % mirror padding
               dist4 = (i-tail_row_index);
               row_padded_nhood(i,:)= col_padded_nhood(tail_row_index-(dist4-1),:);
           end
       else
           row_padded_nhood(i,:)= col_padded_nhood(i,:);
       end
end
 
% ----------------- end  row  padding  -------------------------
 
% ----------------------------------------------------------------
%                    4. assign output  
% ----------------------------------------------------------------
 
if (OUTFORMAT==2)
    %output is a matrix
    y = row_padded_nhood;
else
    %output must be reshaped to a vector
    y = reshape(row_padded_nhood,NH_ROWS * NH_COLS,1);
end
 
% ----------------- assign output   ----------------------------
 
% ----------------------------------------------------------------
%                    5. update persistent variables 
% ----------------------------------------------------------------
 
%  ###  5.1 shift registers (for storing old data_in) ### 
 old_cols = [old_cols(:,2:NH_COLS-1) columnIn];
 
%   ### 5.2 row index register  ### 
% the row index register will latches the value of the row index
% when the count after last column was zero - this helps 
% row padding in case of insufficient or no horizontal blanking
% it is particularly important for the bottom edge of the image. 
max_calc_count = floor(NH_COLS/2);
if int(count_after_last_col)==0 || int(count_after_last_col) == ...
        max_calc_count
    row_index_reg (:)= rowIndex;
end
 
 
% ##   5.3 count after last column  ### 
% it starts after at the next clock after the last column 
% has be received with 1. it goes from 1 to max_calc_count and then to 
% zero. It stays on zero until next last column arrives. 
count_WL= ceil(log2 (max_calc_count))+1;
if int(colIndex)== int(frameSize(2))-1 &&  activePixel   
    count_after_last_col= fi(1,0,count_WL,0);
elseif count_after_last_col == max_calc_count
    count_after_last_col =  fi(0,0,count_WL,0);
elseif count_after_last_col < max_calc_count && count_after_last_col>0          
    count_after_last_col= fi(int(count_after_last_col)+1,0,count_WL,0);     
end

== matlab function fil_videosharp_sim/Frame to Stream/Produce Row-Major Organized Output (Dimensions will be flipped)1 ==
  data: u input; y output; isInputRowMajor parameter
function y = condTranspose(u, isInputRowMajor)
%#eml

if (isInputRowMajor)
    y = u;
else
    y = permute(u,[2,1]);
end

== matlab function fil_videosharp_sim/Frame to Stream/Produce Row-Major Organized Output (Dimensions will be flipped)2 ==
  data: u input; y output; isInputRowMajor parameter
function y = condTranspose(u, isInputRowMajor)
%#eml

if (isInputRowMajor)
    y = u;
else
    y = permute(u,[2,1]);
end
